simulink model "DCmotor"  (R2025b)
settings: Solver=VariableStepAuto  StartTime=0.0  StopTime=2000  RelTol=1e-3
undefined symbols (not defined in the file): alpha_max, beta, d, En, g, Ie, Imaxn, J, Kb_m, KiA, KiE, KiM, KpA, KpE, KpM, Ks, La, Le, m, Ra, Re, rho, Te_max, Te_min, tG_a, tG_e, V, Ve
libraries: slpidlib x3, simulink x1
settings Model: Creator=samug  LastModifiedBy=teocava
settings SolverCC: ZeroCrossAlgorithm=Adaptive
settings DebuggingCC: IgnoredZcDiagnostic=none

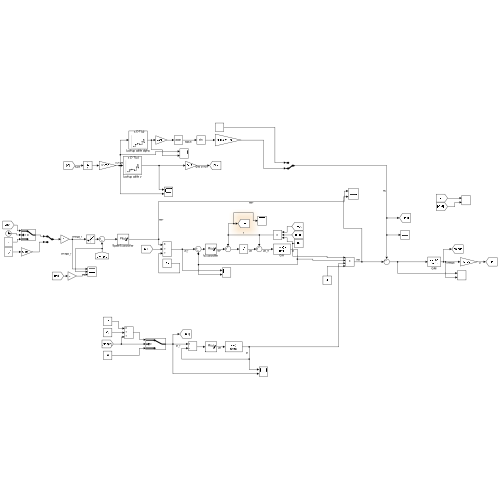
[thumbnail: Simulink's stored preview of the top-level diagram]
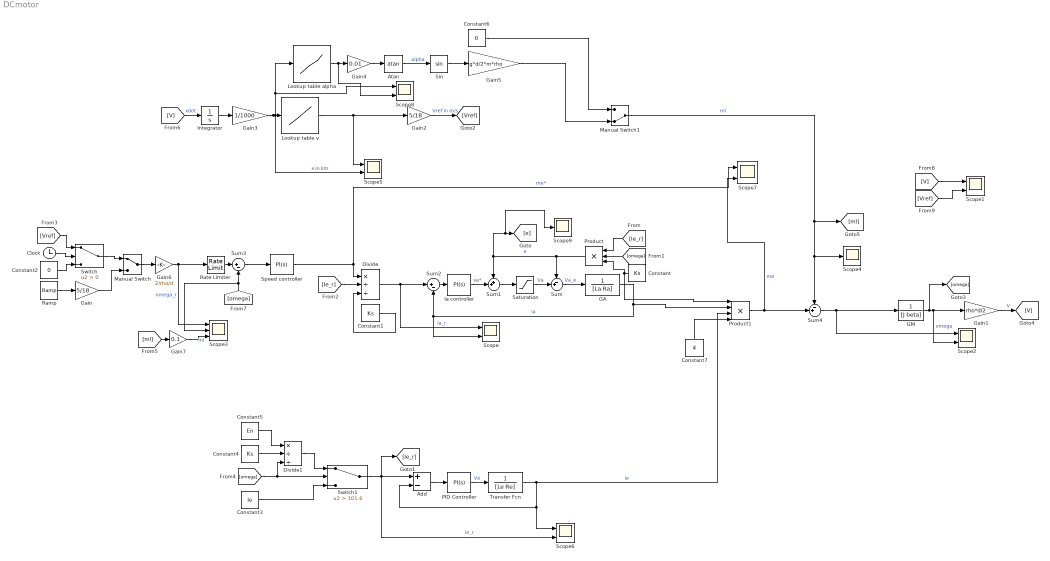
== system DCmotor ==
  Add : Sum  Inputs=+-
  Atan : Trigonometry  Operator=atan
  Clock : Clock
  Constant : Constant  Value=Ks
  Constant1 : Constant  Value=Ks
  Constant2 : Constant  Value=0
  Constant3 : Constant  Value=Ie
  Constant4 : Constant  Value=Ks
  Constant5 : Constant  Value=En
  Constant6 : Constant  Value=0
  Constant7 : Constant  Value=4
  Divide : Product  Inputs=*//
  Divide1 : Product  Inputs=*//
  GA : TransferFcn  Denominator=[La Ra]
  GM : TransferFcn  Denominator=[J beta]
  Gain : Gain  Gain=5/18
  Gain1 : Gain  Gain=rho*d/2
  Gain2 : Gain  Gain=5/18
  Gain3 : Gain  Gain=1/1000
  Gain4 : Gain  Gain=0.01
  Gain5 : Gain  Gain=g*d/2*m*rho
  Gain6 : Gain  Gain=2/rho/d
  Gain7 : Gain  Gain=0.1
  Ia controller : slpidlib/PID Controller  Controller=PI  Form=Parallel  TimeDomain=Continuous-time  UseExternalTs=off  SampleTime=-1  IntegratorMethod=Forward Euler  FilterMethod=Forward Euler  ControllerParametersSource=internal  P=KpA  I=KiA  UseKiTs=off  D=0  UseExternalDerivativeSource=off  N=100  UseFilter=on  TunerSelectOption=Transfer Function Based (PID Tuner App)  InitialConditionSource=internal  InitialConditionForIntegrator=0  InitialConditionForFilter=0  DifferentiatorICPrevScaledInput=0  ExternalReset=none  TrackingMode=off  Kt=1  LimitOutput=on  SatLimitsSource=internal  UpperSaturationLimit=Imaxn  LowerSaturationLimit=-Imaxn  LinearizeAsGain=on  AntiWindupMode=back-calculation  Kb=1/tG_a  LimitIntegrator=off  UpperIntegratorSaturationLimit=inf  LowerIntegratorSaturationLimit=-inf  POutMin=[]  POutMax=[]  IOutMin=[]  IOutMax=[]  DOutMin=[]  DOutMax=[]  NOutMin=[]  NOutMax=[]  SumOutMin=[]  SumOutMax=[]  SaturationOutMin=[]  SaturationOutMax=[]  PParamMin=[]  PParamMax=[]  IParamMin=[]  IParamMax=[]  DParamMin=[]  DParamMax=[]  NParamMin=[]  NParamMax=[]  KbParamMin=[]  KbParamMax=[]  KtParamMin=[]  KtParamMax=[]  KbOutMin=[]  KbOutMax=[]  KtOutMin=[]  KtOutMax=[]  IntegratorOutMin=[]  IntegratorOutMax=[]  FilterOutMin=[]  FilterOutMax=[]  SumI1OutMin=[]  SumI1OutMax=[]  SumI2OutMin=[]  SumI2OutMax=[]  SumI3OutMin=[]  SumI3OutMax=[]  SumI4OutMin=[]  SumI4OutMax=[]  SumDOutMin=[]  SumDOutMax=[]  DifferentiatorOutMin=[]  DifferentiatorOutMax=[]  FilterDiffOutCoefMin=[]  FilterDiffOutCoefMax=[]  ReciprocalOutMin=[]  ReciprocalOutMax=[]  SumDenOutMin=[]  SumDenOutMax=[]  SumNumOutMin=[]  SumNumOutMax=[]  DivideOutMin=[]  DivideOutMax=[]  UdiffTsProdOutMin=[]  UdiffTsProdOutMax=[]  NTsProdOutMin=[]  NTsProdOutMax=[]  UintegralTsProdOutMin=[]  UintegralTsProdOutMax=[]  UngainTsProdOutMin=[]  UngainTsProdOutMax=[]  ClampingZeroOutDataTypeStr=Inherit: Inherit via back propagation  ClampingZeroOutMin=[]  ClampingZeroOutMax=[]  FilterDenConstantOutDataTypeStr=Inherit: Inherit via back propagation  FilterDenConstantOutMin=[]  FilterDenConstantOutMax=[]  PCopyOutDataTypeStr=Inherit: Inherit via back propagation  PCopyOutMin=[]  PCopyOutMax=[]  NCopyOutDataTypeStr=Inherit: Inherit via back propagation  NCopyOutMin=[]  NCopyOutMax=[]  IntegratorContinuousStateAttributes=''  IntegratorStateMustResolveToSignalObject=off  IntegratorRTWStateStorageClass=Auto  FilterContinuousStateAttributes=''  FilterStateMustResolveToSignalObject=off  FilterRTWStateStorageClass=Auto  ParallelPVariant=InternalParameters  IdealPVariant=Disabled  IVariant=InternalParameters  DVariant=Disabled  IntegratorVariant=Continuous  SatVariant=Enabled  AWVariant=BackCalculation  PCopyVariant=Disabled  TRVariant=Disabled  FdbkBlocksVariant=Forward  IdealPFdbkVariant=Disabled  SatFdbkVariant=Disabled  DerivativeFilterVariant=Disabled  NVariant=Disabled  NCopyVariant=Disabled_SignalSpec  FilterICVariant=Disabled  IntegratorICVariant=InternalICs  ExternalResetVariant=Disabled  TRSumVariant=Passthrough  SumFdbkVariant=Disabled  SumVariant=Sum_PI  TsampFilterVariant=InternalTs  TsampNgainVariant=Passthrough  TsampIntegralVariant=Disabled_SignalSpec  ExternalSaturationOutDataTypeStr=Inherit: Same as second input  DerivativeSourceVariant=Disabled  PreIntVariant=InternalPreInt
  Integrator : Integrator
  Lookup table alpha : Lookup_n-D  NumberOfTableDimensions=1  BreakpointsForDimension1=[0;1;2;3;3.5;4;6;7;8;8.5;9;10]  Table=[0;0;0;5;5;0;0;0;-5;-5;0;0]  InterpMethod=Flat  InternalRulePriority=Speed  RndMeth=Simplest
  Lookup table v : Lookup_n-D  NumberOfTableDimensions=1  BreakpointsForDimension1=[0;0.90000000000000002;1;2.8999999999999999;3;3.8999999999999999;4;5.9000000000000004;6;7.9000000000000004;8;8.9000000000000004;9;10]  Table=[10.921;10.921;21.8421;21.8421;21.8421;21.8421;42;42;21.8421;21.8421;21.8421;21.8421;10.921;10.921]  InterpMethod=Flat  InternalRulePriority=Speed  RndMeth=Simplest
  Manual Switch : ManualSwitch
  Manual Switch1 : ManualSwitch  CurrentSetting=0
  PID Controller : slpidlib/PID Controller  Controller=PI  Form=Parallel  TimeDomain=Continuous-time  UseExternalTs=off  SampleTime=-1  IntegratorMethod=Forward Euler  FilterMethod=Forward Euler  ControllerParametersSource=internal  P=KpE  I=KiE  UseKiTs=off  D=0  UseExternalDerivativeSource=off  N=100  UseFilter=on  TunerSelectOption=Transfer Function Based (PID Tuner App)  InitialConditionSource=internal  InitialConditionForIntegrator=0  InitialConditionForFilter=0  DifferentiatorICPrevScaledInput=0  ExternalReset=none  TrackingMode=off  Kt=1  LimitOutput=on  SatLimitsSource=internal  UpperSaturationLimit=Ve  LowerSaturationLimit=-Ve  LinearizeAsGain=on  AntiWindupMode=back-calculation  Kb=1/tG_e  LimitIntegrator=off  UpperIntegratorSaturationLimit=inf  LowerIntegratorSaturationLimit=-inf  POutMin=[]  POutMax=[]  IOutMin=[]  IOutMax=[]  DOutMin=[]  DOutMax=[]  NOutMin=[]  NOutMax=[]  SumOutMin=[]  SumOutMax=[]  SaturationOutMin=[]  SaturationOutMax=[]  PParamMin=[]  PParamMax=[]  IParamMin=[]  IParamMax=[]  DParamMin=[]  DParamMax=[]  NParamMin=[]  NParamMax=[]  KbParamMin=[]  KbParamMax=[]  KtParamMin=[]  KtParamMax=[]  KbOutMin=[]  KbOutMax=[]  KtOutMin=[]  KtOutMax=[]  IntegratorOutMin=[]  IntegratorOutMax=[]  FilterOutMin=[]  FilterOutMax=[]  SumI1OutMin=[]  SumI1OutMax=[]  SumI2OutMin=[]  SumI2OutMax=[]  SumI3OutMin=[]  SumI3OutMax=[]  SumI4OutMin=[]  SumI4OutMax=[]  SumDOutMin=[]  SumDOutMax=[]  DifferentiatorOutMin=[]  DifferentiatorOutMax=[]  FilterDiffOutCoefMin=[]  FilterDiffOutCoefMax=[]  ReciprocalOutMin=[]  ReciprocalOutMax=[]  SumDenOutMin=[]  SumDenOutMax=[]  SumNumOutMin=[]  SumNumOutMax=[]  DivideOutMin=[]  DivideOutMax=[]  UdiffTsProdOutMin=[]  UdiffTsProdOutMax=[]  NTsProdOutMin=[]  NTsProdOutMax=[]  UintegralTsProdOutMin=[]  UintegralTsProdOutMax=[]  UngainTsProdOutMin=[]  UngainTsProdOutMax=[]  ClampingZeroOutDataTypeStr=Inherit: Inherit via back propagation  ClampingZeroOutMin=[]  ClampingZeroOutMax=[]  FilterDenConstantOutDataTypeStr=Inherit: Inherit via back propagation  FilterDenConstantOutMin=[]  FilterDenConstantOutMax=[]  PCopyOutDataTypeStr=Inherit: Inherit via back propagation  PCopyOutMin=[]  PCopyOutMax=[]  NCopyOutDataTypeStr=Inherit: Inherit via back propagation  NCopyOutMin=[]  NCopyOutMax=[]  IntegratorContinuousStateAttributes=''  IntegratorStateMustResolveToSignalObject=off  IntegratorRTWStateStorageClass=Auto  FilterContinuousStateAttributes=''  FilterStateMustResolveToSignalObject=off  FilterRTWStateStorageClass=Auto  ParallelPVariant=InternalParameters  IdealPVariant=Disabled  IVariant=InternalParameters  DVariant=Disabled  IntegratorVariant=Continuous  SatVariant=Enabled  AWVariant=BackCalculation  PCopyVariant=Disabled  TRVariant=Disabled  FdbkBlocksVariant=Forward  IdealPFdbkVariant=Disabled  SatFdbkVariant=Disabled  DerivativeFilterVariant=Disabled  NVariant=Disabled  NCopyVariant=Disabled_SignalSpec  FilterICVariant=Disabled  IntegratorICVariant=InternalICs  ExternalResetVariant=Disabled  TRSumVariant=Passthrough  SumFdbkVariant=Disabled  SumVariant=Sum_PI  TsampFilterVariant=InternalTs  TsampNgainVariant=Passthrough  TsampIntegralVariant=Disabled_SignalSpec  ExternalSaturationOutDataTypeStr=Inherit: Same as second input  DerivativeSourceVariant=Disabled  PreIntVariant=InternalPreInt
  Product : Product  Inputs=3
  Product1 : Product  Inputs=4
  Ramp : simulink/Sources/Ramp  slope=1  start=0  InitialOutput=0
  Rate Limiter : RateLimiter  RisingSlewLimit=alpha_max  FallingSlewLimit=-alpha_max  SampleTimeMode=inherited
  Saturation : Saturate  UpperLimit=V  LowerLimit=-V
  Scope{,1..2,5..8} (7 alike) : Scope  NumInputPorts=2
      Scope settings: ActiveDisplayYMinimum=-159.48999663477295  ActiveDisplayYMaximum=185.64177035527743
      Scope1 settings: ActiveDisplayYMinimum=-1.4643256464099137  ActiveDisplayYMaximum=13.178930817689226
      Scope2 settings: ActiveDisplayYMinimum=-3330.8125193103629  ActiveDisplayYMaximum=3317.4867325649752  DataLoggingVariableName=ScopeData2
      Scope5 settings: ActiveDisplayYMinimum=-1  ActiveDisplayYMaximum=1  DataLoggingVariableName=ScopeData5
      Scope6 settings: ActiveDisplayYMinimum=-0.67260675095632072  ActiveDisplayYMaximum=5.6460015838161812  DataLoggingVariableName=ScopeData6
      Scope7 settings: ActiveDisplayYMinimum=-3164.6276859947629  ActiveDisplayYMaximum=3206.4148145983472  DataLoggingVariableName=ScopeData7
      Scope8 settings: ActiveDisplayYMinimum=-1  ActiveDisplayYMaximum=1  DataLoggingVariableName=ScopeData8
  Scope3 : Scope  NumInputPorts=3
      settings: ActiveDisplayYMinimum=-105.59296  ActiveDisplayYMaximum=609.01437  DataLoggingVariableName=ScopeData3
  Scope4 : Scope
      settings: ActiveDisplayYMinimum=-928.08589  ActiveDisplayYMaximum=928.08589  DataLoggingVariableName=ScopeData4
  Scope9 : Scope
      settings: ActiveDisplayYMinimum=-1  ActiveDisplayYMaximum=1
  Sin : Trigonometry
  Speed controller : slpidlib/PID Controller  Controller=PI  Form=Parallel  TimeDomain=Continuous-time  UseExternalTs=off  SampleTime=-1  IntegratorMethod=Forward Euler  FilterMethod=Forward Euler  ControllerParametersSource=internal  P=KpM  I=KiM  UseKiTs=off  D=0  UseExternalDerivativeSource=off  N=100  UseFilter=on  TunerSelectOption=Transfer Function Based (PID Tuner App)  InitialConditionSource=internal  InitialConditionForIntegrator=0  InitialConditionForFilter=0  DifferentiatorICPrevScaledInput=0  ExternalReset=none  TrackingMode=off  Kt=1  LimitOutput=on  SatLimitsSource=internal  UpperSaturationLimit=Te_max  LowerSaturationLimit=Te_min  LinearizeAsGain=on  AntiWindupMode=back-calculation  Kb=Kb_m  LimitIntegrator=off  UpperIntegratorSaturationLimit=inf  LowerIntegratorSaturationLimit=-inf  POutMin=[]  POutMax=[]  IOutMin=[]  IOutMax=[]  DOutMin=[]  DOutMax=[]  NOutMin=[]  NOutMax=[]  SumOutMin=[]  SumOutMax=[]  SaturationOutMin=[]  SaturationOutMax=[]  PParamMin=[]  PParamMax=[]  IParamMin=[]  IParamMax=[]  DParamMin=[]  DParamMax=[]  NParamMin=[]  NParamMax=[]  KbParamMin=[]  KbParamMax=[]  KtParamMin=[]  KtParamMax=[]  KbOutMin=[]  KbOutMax=[]  KtOutMin=[]  KtOutMax=[]  IntegratorOutMin=[]  IntegratorOutMax=[]  FilterOutMin=[]  FilterOutMax=[]  SumI1OutMin=[]  SumI1OutMax=[]  SumI2OutMin=[]  SumI2OutMax=[]  SumI3OutMin=[]  SumI3OutMax=[]  SumI4OutMin=[]  SumI4OutMax=[]  SumDOutMin=[]  SumDOutMax=[]  DifferentiatorOutMin=[]  DifferentiatorOutMax=[]  FilterDiffOutCoefMin=[]  FilterDiffOutCoefMax=[]  ReciprocalOutMin=[]  ReciprocalOutMax=[]  SumDenOutMin=[]  SumDenOutMax=[]  SumNumOutMin=[]  SumNumOutMax=[]  DivideOutMin=[]  DivideOutMax=[]  UdiffTsProdOutMin=[]  UdiffTsProdOutMax=[]  NTsProdOutMin=[]  NTsProdOutMax=[]  UintegralTsProdOutMin=[]  UintegralTsProdOutMax=[]  UngainTsProdOutMin=[]  UngainTsProdOutMax=[]  ClampingZeroOutDataTypeStr=Inherit: Inherit via back propagation  ClampingZeroOutMin=[]  ClampingZeroOutMax=[]  FilterDenConstantOutDataTypeStr=Inherit: Inherit via back propagation  FilterDenConstantOutMin=[]  FilterDenConstantOutMax=[]  PCopyOutDataTypeStr=Inherit: Inherit via back propagation  PCopyOutMin=[]  PCopyOutMax=[]  NCopyOutDataTypeStr=Inherit: Inherit via back propagation  NCopyOutMin=[]  NCopyOutMax=[]  IntegratorContinuousStateAttributes=''  IntegratorStateMustResolveToSignalObject=off  IntegratorRTWStateStorageClass=Auto  FilterContinuousStateAttributes=''  FilterStateMustResolveToSignalObject=off  FilterRTWStateStorageClass=Auto  ParallelPVariant=InternalParameters  IdealPVariant=Disabled  IVariant=InternalParameters  DVariant=Disabled  IntegratorVariant=Continuous  SatVariant=Enabled  AWVariant=BackCalculation  PCopyVariant=Disabled  TRVariant=Disabled  FdbkBlocksVariant=Forward  IdealPFdbkVariant=Disabled  SatFdbkVariant=Disabled  DerivativeFilterVariant=Disabled  NVariant=Disabled  NCopyVariant=Disabled_SignalSpec  FilterICVariant=Disabled  IntegratorICVariant=InternalICs  ExternalResetVariant=Disabled  TRSumVariant=Passthrough  SumFdbkVariant=Disabled  SumVariant=Sum_PI  TsampFilterVariant=InternalTs  TsampNgainVariant=Passthrough  TsampIntegralVariant=Disabled_SignalSpec  ExternalSaturationOutDataTypeStr=Inherit: Same as second input  DerivativeSourceVariant=Disabled  PreIntVariant=InternalPreInt
  Sum : Sum  Inputs=-+|
  Sum1 : Sum  Inputs=++|
  Sum2 : Sum  Inputs=|+-
  Sum3 : Sum  Inputs=|+-
  Sum4 : Sum  Inputs=-+|
  Switch : Switch  Criteria=u2 > Threshold  SaturateOnIntegerOverflow=off  InputSameDT=off
  Switch1 : Switch  Criteria=u2 > Threshold  Threshold=101.6  SaturateOnIntegerOverflow=off  InputSameDT=off
  Transfer Fcn : TransferFcn  Denominator=[Le Re]
  wires:
  Sum/1 -> GA/1  "Va_e"
  Saturation/1 -> Sum/2  "Va"
  Sum1/1 -> Saturation/1
  Ia controller/1 -> Sum1/2  "va*"
  Sum2/1 -> Ia controller/1
  GA/1 -> Scope/2, Sum2/2, Product1/2  "ia"
  Divide/1 -> Sum2/1, Scope/1  "ia_r"
  Product/1 -> Sum/1, Sum1/1, Scope9/1, [e]  "e"
  [Ie_r] -> Product/1
  [omega] -> Product/2
  Constant/1 -> Product1/1, Product/3
  [Ie_r] -> Divide/2
  Constant1/1 -> Divide/3
  Speed controller/1 -> Scope7/1, Divide/1  "me*"
  Sum3/1 -> Speed controller/1
  Switch/1 -> Manual Switch/1
  Gain/1 -> Manual Switch/2
  Ramp/1 -> Gain/1
  Constant2/1 -> Switch/3
  Clock/1 -> Switch/2
  [Vref] -> Switch/1
  GM/1 -> [omega], Scope2/2, Gain1/1  "omega"
  Divide1/1 -> Switch1/1
  Constant3/1 -> Switch1/3
  Switch1/1 -> Scope6/2, Add/1, [Ie_r]  "ie_r"
  Add/1 -> PID Controller/1
  PID Controller/1 -> Transfer Fcn/1  "Ve"
  Transfer Fcn/1 -> Add/2, Scope6/1, Product1/3  "ie"
  Constant4/1 -> Divide1/2
  Constant5/1 -> Divide1/1
  Gain2/1 -> [Vref]  "Vref in m/s"
  [V] -> Integrator/1  "xdot"
  Integrator/1 -> Gain3/1
  Gain3/1 -> Scope5/2, Scope8/1, Lookup table alpha/1, Lookup table v/1  "x in km"
  Lookup table alpha/1 -> Scope8/2, Gain4/1
  Gain4/1 -> Atan/1
  Atan/1 -> Sin/1  "alpha"
  Sin/1 -> Gain5/1
  Gain5/1 -> Manual Switch1/2
  Constant6/1 -> Manual Switch1/1
  [omega] -> Scope3/2, Sum3/2
  Product1/1 -> Sum4/2, Scope7/2  "me"
  Sum4/1 -> Scope2/1, GM/1
  Manual Switch1/1 -> [ml], Scope4/1, Sum4/1  "ml"
  [V] -> Scope1/1
  [Vref] -> Scope1/2
  Manual Switch/1 -> Gain6/1
  Gain6/1 -> Scope3/1, Rate Limiter/1  "omega_r"
  Gain1/1 -> [V]  "V"
  Constant7/1 -> Product1/4
  [ml] -> Gain7/1
  Gain7/1 -> Scope3/3  "ml"
  [omega] -> Divide1/3, Switch1/2
  Lookup table v/1 -> Scope5/1, Gain2/1
  Rate Limiter/1 -> Sum3/1
